simulink model "dryden"  (R2019b)
settings: Solver=VariableStepAuto  StartTime=0.0  StopTime=10.0  RelTol=1e-3
values from neighbouring files (symbols this model uses):
  attitude = Rzyx(0,0,0)    [run_dryden.m]
  height = 10000    [run_dryden.m]
  q = table(:,2:5)    [attitude (1).m]    (also in kinematics_quaternion.m = zeros(N,4))
  speed = 25    [run_dryden.m]
undefined symbols (not defined in the file or in its folder): F, MIL
libraries: aerolibwind2 x1
settings Model: Creator=hakonhhe  LastModifiedBy=hakonhhe

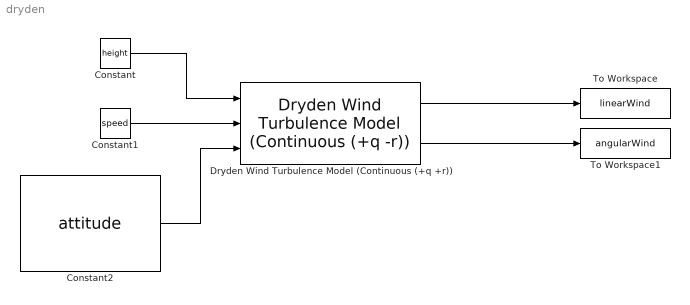
== system dryden ==
  Constant : Constant  Value=height
  Constant1 : Constant  Value=speed
  Constant2 : Constant  Value=attitude  VectorParams1D=off
  Dryden Wind Turbulence Model (Continuous (+q +r)) : aerolibwind2/Dryden Wind Turbulence Model  (Continuous (+q -r))  units=Metric (MKS)  spec=MIL-F-8785C  model=Continuous Dryden (+q +r)  W20=10  Wdeg=90  TurbProb=10^-4  L_high=533.4  Wingspan=10  ts=0.1  Seed=[23341 23342 23343 23344]  T_on=on
      settings: SourceProductName=Aerospace Blockset
  To Workspace : ToWorkspace  VariableName=linearWind  SaveFormat=Timeseries  SampleTime=-1
  To Workspace1 : ToWorkspace  VariableName=angularWind  SaveFormat=Timeseries  SampleTime=-1
  wires:
  Constant/1 -> Dryden Wind Turbulence Model (Continuous (+q +r))/1
  Constant1/1 -> Dryden Wind Turbulence Model (Continuous (+q +r))/2
  Dryden Wind Turbulence Model (Continuous (+q +r))/1 -> To Workspace/1
  Dryden Wind Turbulence Model (Continuous (+q +r))/2 -> To Workspace1/1
  Constant2/1 -> Dryden Wind Turbulence Model (Continuous (+q +r))/3
